simulink library "Actuator_AC_Lib"  (R2014a)
settings: Solver=ode45  StartTime=0.0  StopTime=10.0  RelTol=1e-3
undefined symbols (not defined in the file): APN_Param, DiscIntNeverNeededParam, driveGuiManager, gcbh
libraries: powerlib x14, Actuator_AC_Lib x3, AC6DriveInternalModels x3, simulink x3, DriveInternalModels x1, Lamp_Lib x1
Description:
  | Copyright 2014 The MathWorks, Inc.
settings Model: Creator=smiller  LastModifiedBy=psanghvi

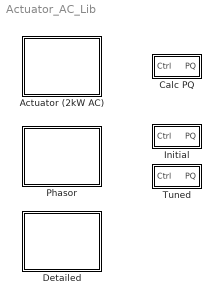
== system Actuator_AC_Lib ==
  Actuator (2kW AC) : Subsystem  BlockChoice=Detailed
      settings: TemplateBlock=self  MemberBlocks=Detailed,Phasor
  Calc PQ : Subsystem  BlockChoice=Initial
      settings: TemplateBlock=self  MemberBlocks=Initial,Tuned
  Detailed : Subsystem
      mask Display: image(imread('ActuatorAC_Detailed_IMAGE.jpg'));
  Initial : Subsystem
  Phasor : Subsystem
      mask Display: image(imread('ActuatorAC_Phasor_IMAGE.jpg'));
  Tuned : Subsystem

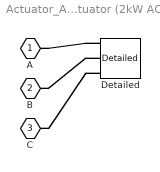
== system Actuator_AC_Lib/Actuator (2kW AC) ==
  Detailed : Actuator_AC_Lib/Detailed  SystemSampleTime=-1
  A : PMIOPort  Port=1  Side=Left
  B : PMIOPort  Port=2  Side=Left
  C : PMIOPort  Port=3  Side=Left
  connections:
  Detailed/LConn1 -- A/RConn1
  Detailed/LConn2 -- B/RConn1
  Detailed/LConn3 -- C/RConn1

== system Actuator_AC_Lib/Calc PQ ==
  Ctrl : Inport
  Initial : Actuator_AC_Lib/Initial
  PQ : Outport
  wires:
  Ctrl/1 -> Initial/1
  Initial/1 -> PQ/1

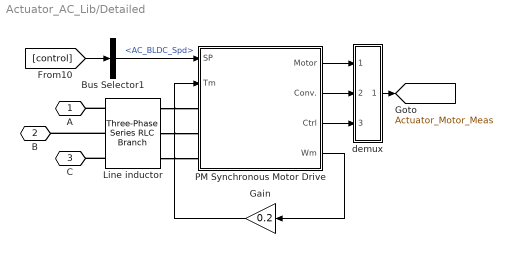
== system Actuator_AC_Lib/Detailed ==
  Bus Selector1 : BusSelector  OutputSignals=AC_BLDC_Spd
  Gain : Gain  Gain=0.2
  Line inductor : powerlib/Elements/Three-Phase Series RLC Branch  LConnTagsString=A|B|C  RConnTagsString=A|B|C  BranchType=L  Resistance=[]  Inductance=1e-3  Capacitance=[]  Measurements=None
  PM Synchronous Motor Drive : Subsystem  LoadFcn=driveGuiManager('Load',get_param(gcb,'driveType'), gcbh);  mask(PM Synchronous Motor Drive){AverageValue=on, MechanicalLoad=Torque Tm, driveType=AC6}
      mask prompts: AverageValue "Average value model"; MechanicalLoad "Mechanical input:"; driveType "Drive type:"
      mask init:
      | block = gcbh;
      | [X1,X1m,X2,X2m,X3,X4,Y1,Y1m,Y2,Y2m,Y3,Y4,color1,color2]=spsdrivelogo;
      | Ts = drivelibInitSampleTime(block);    
      | driveGuiManager('Siminit',driveType,block);
      | SetInternalDriveModel(driveType,AverageValue,block);
      | setInternalDriveMechInput(driveType,getfullname(block));
      | power_initmask();
      settings: DeleteFcn="driveGuiManager('Delete',get_param(gcb,'driveType')  ,gcbh)"  CloseFcn="driveGuiManager('Delete',get_param(gcb,'driveType')  ,gcbh)"  ParentCloseFcn="driveGuiManager('Hide',get_param(gcb,'driveType')  ,gcbh)"
      settings: OpenFcn=|
      | if (power_openblockproxy ('secondary'))
      | driveGuiManager('Create',get_param(gcb,'driveType')  ,gcbh)
      | end;
      mask Help: web(psbhelp)
      mask TypeOptions MechanicalLoad: Torque Tm | Speed w
      mask TypeOptions driveType: AC6
      mask Display:
      | patch([X1 X1m],[Y1 Y1m],color1);
      | patch(X3,Y3,color2);
      | plot([X1 X1m X2 X2m X3 X4],[Y1 Y1m Y2 Y2m Y3 Y4]);
      | text(0.5,0.3,'AC6','HorizontalAlignment','center')
  demux : Subsystem
  A : PMIOPort  Port=1  Side=Left
  B : PMIOPort  Port=2  Side=Left
  C : PMIOPort  Port=3  Side=Left
  tag scope: Actuator_Motor_Meas=global
  wires:
  PM Synchronous Motor Drive/3(Ctrl) -> demux/3(Ctrl)
  PM Synchronous Motor Drive/2(Conv.) -> demux/2(Conv.)
  PM Synchronous Motor Drive/1(Motor) -> demux/1(motor)
  PM Synchronous Motor Drive/4(Wm) -> Gain/1
  Gain/1 -> PM Synchronous Motor Drive/2(Tm)
  Bus Selector1/1 -> PM Synchronous Motor Drive/1(SP)  "<AC_BLDC_Spd>"
  demux/1(S) -> [Actuator_Motor_Meas]
  [control] -> Bus Selector1/1
  connections:
  Line inductor/LConn1 -- A/RConn1
  Line inductor/LConn2 -- B/RConn1
  Line inductor/LConn3 -- C/RConn1
  Line inductor/RConn1 -- PM Synchronous Motor Drive/LConn1
  Line inductor/RConn2 -- PM Synchronous Motor Drive/LConn2
  Line inductor/RConn3 -- PM Synchronous Motor Drive/LConn3

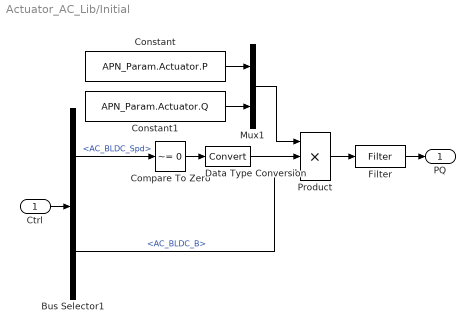
== system Actuator_AC_Lib/Initial ==
  Ctrl : Inport
  Bus Selector1 : BusSelector  OutputSignals=AC_BLDC_Spd,AC_BLDC_B
  Compare To Zero : simulink/Logic and Bit Operations/Compare To Zero  relop=~=  OutDataTypeStr=boolean
  Constant : Constant  Value=APN_Param.Actuator.P
  Constant1 : Constant  Value=APN_Param.Actuator.Q
  Data Type Conversion : DataTypeConversion
  Filter : Lamp_Lib/Initial/Filter  b=1e-2  x_initial=[APN_Param.Actuator.P APN_Param.Actuator.Q]*0
  Mux1 : Mux  Inputs=2
  Product : Product  Inputs=3
  PQ : Outport
  wires:
  Filter/1 -> PQ/1
  Bus Selector1/2 -> Product/3  "<AC_BLDC_B>"
  Bus Selector1/1 -> Compare To Zero/1  "<AC_BLDC_Spd>"
  Ctrl/1 -> Bus Selector1/1
  Compare To Zero/1 -> Data Type Conversion/1
  Data Type Conversion/1 -> Product/2
  Mux1/1 -> Product/1
  Constant/1 -> Mux1/1
  Constant1/1 -> Mux1/2
  Product/1 -> Filter/1

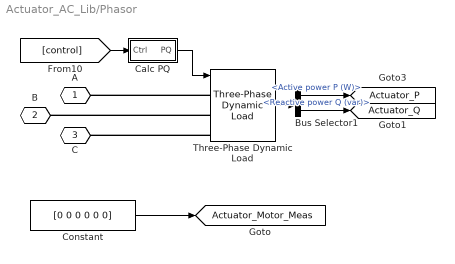
== system Actuator_AC_Lib/Phasor ==
  Bus Selector1 : BusSelector  OutputSignals=Active power P (W),Reactive power Q (var)
  Calc PQ : Subsystem  BlockChoice=Initial
      settings: AttributesFormatString=%<BlockChoice>  TemplateBlock=Actuator_AC_Lib/Calc PQ  MemberBlocks=Initial,Tuned
  Constant : Constant  Value=[0 0 0 0 0 0]
  Three-Phase Dynamic Load : powerlib/Elements/Three-Phase Dynamic Load  NominalVoltage=[ 500e3 400 ]  ActiveReactivePowers=[APN_Param.Actuator.P APN_Param.Actuator.Q]  PositiveSequence=[0.0004 0]  ExternalControl=on  NpNq=[1.3 2]  TimeConstants="[0  0  0  0]"  MinimumVoltage=0.7  LoadFlowParameters=[4,0,0,0,0]
  A : PMIOPort  Port=1  Side=Right
  B : PMIOPort  Port=2  Side=Right
  C : PMIOPort  Port=3  Side=Right
  tag scope: Actuator_Motor_Meas=global, Actuator_P=global, Actuator_Q=global
  wires:
  Bus Selector1/1 -> [Actuator_P]  "<Active power P (W)>"
  Three-Phase Dynamic Load/1 -> Bus Selector1/1
  Calc PQ/1(PQ) -> Three-Phase Dynamic Load/1
  Constant/1 -> [Actuator_Motor_Meas]
  Bus Selector1/2 -> [Actuator_Q]  "<Reactive power Q (var)>"
  [control] -> Calc PQ/1(Ctrl)
  connections:
  Three-Phase Dynamic Load/LConn3 -- C/RConn1
  Three-Phase Dynamic Load/LConn1 -- A/RConn1
  Three-Phase Dynamic Load/LConn2 -- B/RConn1

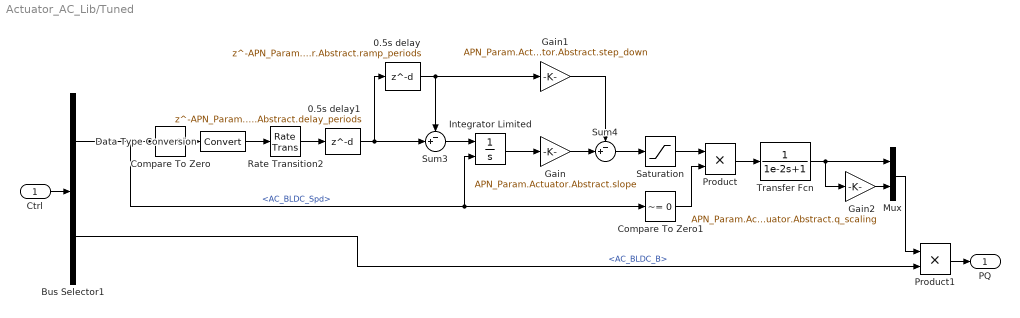
== system Actuator_AC_Lib/Tuned ==
  Ctrl : Inport
  0.5s delay : Delay  DelayLength=APN_Param.Actuator.Abstract.ramp_periods  SampleTime=0.01
  0.5s delay1 : Delay  DelayLength=APN_Param.Actuator.Abstract.delay_periods  SampleTime=0.01
  Bus Selector1 : BusSelector  OutputSignals=AC_BLDC_Spd,AC_BLDC_B
  Compare To Zero : simulink/Logic and Bit Operations/Compare To Zero  relop=~=  OutDataTypeStr=boolean
  Compare To Zero1 : simulink/Logic and Bit Operations/Compare To Zero  relop=~=  OutDataTypeStr=boolean
  Data Type Conversion : DataTypeConversion
  Gain : Gain  Gain=APN_Param.Actuator.Abstract.slope
  Gain1 : Gain  Gain=APN_Param.Actuator.Abstract.step_down
  Gain2 : Gain  Gain=APN_Param.Actuator.Abstract.q_scaling
  Integrator Limited : Integrator  ExternalReset=falling  LimitOutput=on  UpperSaturationLimit=1  LowerSaturationLimit=0
  Mux : Mux  Inputs=2
  Product : Product
  Product1 : Product
  Rate Transition2 : RateTransition  OutPortSampleTime=0.01
  Saturation : Saturate  UpperLimit=1160  LowerLimit=0
  Sum3 : Sum  Inputs=-+|  SaturateOnIntegerOverflow=on  InputSameDT=on  OutDataTypeStr=Inherit: Same as first input
  Sum4 : Sum  Inputs=-+|  SaturateOnIntegerOverflow=on  InputSameDT=on  OutDataTypeStr=Inherit: Same as first input
  Transfer Fcn : TransferFcn  Denominator=[1e-2 1]
  PQ : Outport
  wires:
  Compare To Zero1/1 -> Product/2
  Saturation/1 -> Product/1
  Sum4/1 -> Saturation/1
  0.5s delay/1 -> Gain1/1, Sum3/1
  Gain1/1 -> Sum4/1
  Product/1 -> Transfer Fcn/1
  Sum3/1 -> Integrator Limited/1
  Rate Transition2/1 -> 0.5s delay1/1
  Gain/1 -> Sum4/2
  Data Type Conversion/1 -> Rate Transition2/1
  Integrator Limited/1 -> Gain/1
  Compare To Zero/1 -> Data Type Conversion/1
  Transfer Fcn/1 -> Gain2/1, Mux/1
  Ctrl/1 -> Bus Selector1/1
  Gain2/1 -> Mux/2
  Mux/1 -> Product1/1
  Bus Selector1/1 -> Integrator Limited/2, Compare To Zero1/1, Compare To Zero/1  "<AC_BLDC_Spd>"
  0.5s delay1/1 -> Sum3/2, 0.5s delay/1
  Bus Selector1/2 -> Product1/2  "<AC_BLDC_B>"
  Product1/1 -> PQ/1

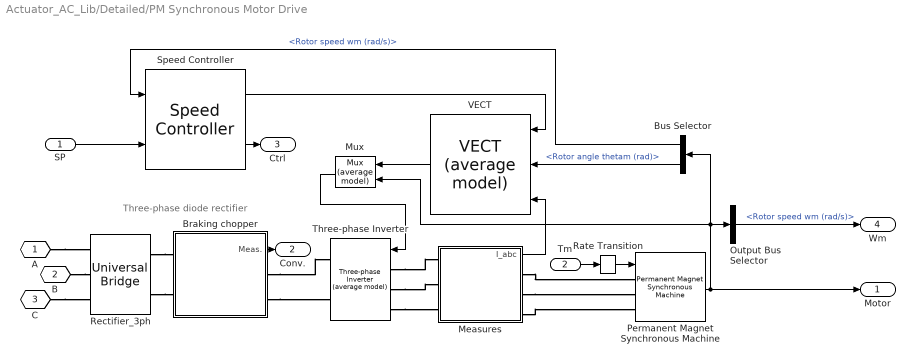
== system Actuator_AC_Lib/Detailed/PM Synchronous Motor Drive ==
  note: Three-phase
      | diode rectifier
  SP : Inport
  Tm : Inport  Port=2
  Braking chopper : Subsystem  StartFcn=|  mask(Braking chopper){chopa=290, chopd=280, freq_chop=4000, cap_bus=2000e-6, br=8}
      | chopa=str2num(get_param(gcb,'chopa'));                                                               
      | chopd=str2num(get_param(gcb,'chopd'));                                                               
      | if (chopa < chopd)                                                                                   
      |     error('Activation voltage must be greater than or equal to shutdown voltage in Braking chopper');
      | end
      mask prompts: chopa "Chopper activation voltage (V)"; chopd "Chopper shutdown voltage (V)"; freq_chop "Braking chopper frequency (Hz)"; cap_bus "DC bus capacitance (F)"; br "Braking resistance (ohms)"
      mask help: This block implement a DC link between the rectifier and the inverter. It also contains a DC bus integrated braking chopper. The braking resistor must be set properly to avoid oscillation.
      mask init:
      | if chopa < chopd;
      |     chopa = chopd;
      | end
      | [X1,X1m,X2,X2m,X3,X4,Y1,Y1m,Y2,Y2m,Y3,Y4,color1,color2]=spsdrivelogo;
      mask Display:
      | patch([X1 X1m],[Y1 Y1m],color1);
      | patch(X3,Y3,color2);
      | plot([X1 X1m X2 X2m X3 X4],[Y1 Y1m Y2 Y2m Y3 Y4]);
  Bus Selector : BusSelector  OutputSignals=Rotor speed wm (rad/s),Rotor angle thetam (rad)
  Measures : Subsystem
  Mux : AC6DriveInternalModels/Mux (average model)
  Output Bus Selector : BusSelector  OutputSignals=Rotor speed wm (rad/s)
  Permanent Magnet Synchronous Machine : powerlib/Machines/Permanent Magnet Synchronous Machine  NbPhases=3  FluxDistribution=Sinusoidal  RotorType=Round  MechanicalLoad=Torque Tm  PresetModel=No  ShowDetailedParameters=on  MeasurementBus=off  Resistance=0.2  Inductance=0  dqInductances=[8.5e-3,8.5e-3]  La=0.000835  MachineConstant=Flux linkage established by magnets (V.s)  Flux=0.175  VoltageCst=126.966  TorqueCst=1.05  Flat=0  Mechanical=[0.089,0.005,4]  PolePairs=4  InitialConditions=[0,0,0,0]  InitialConditions5ph=[0 0 0 0 0 0]  TsPowergui=0  TsBlock=-1  RefAngle=90 degrees behind phase A axis (modified Park)
      settings: AttributesFormatString=\n
  Rate Transition : RateTransition  OutPortSampleTime=Ts
  Rectifier_3ph : powerlib/Power Electronics/Universal Bridge  Arms=3  SnubberResistance=10e3  SnubberCapacitance=20e-9  Device=Diodes  Ron=1e-3  Lon=0  ForwardVoltages="[  0,  0  ]"  ForwardVoltage=1.3  GTOparameters=[ 10e-6, 20e-6 ]  IGBTparameters=[ 1e-6 , 2e-6 ]  Measurements=All voltages and currents  Measurements_2=None  converterType=Rectifier
  Speed Controller : DriveInternalModels/AC drives/Speed Controller AC67/Speed Controller  SwK=Speed regulation  ramp=[-1000,1000]  kp=5  ki=100  fc=100  ctrl_sat=[-50,50]  Tsc=150e-6
  Three-phase Inverter : AC6DriveInternalModels/Three-phase Inverter (average model)  Arms=3  SnubberResistance=5000  SnubberCapacitance=inf  Device=IGBT / Diodes  Ron=1e-3  Lon=0  ForwardVoltages=[0.8,0.8]  ForwardVoltage=0  GTOparameters=[0,0]  IGBTparameters=[1e-6,2e-6]  Measurements=All voltages and currents  converterType=Inverter  SourceFrequency=60  dqInductances=[8.5e-3,8.5e-3]  Flux=0.175  Resistance=0.2  p=4
  VECT : AC6DriveInternalModels/VECT (average model)  nb_p=4  lambda=0.175  freq_max=20e3  Ts_vect=50e-6  h=0.1
  A : PMIOPort  Port=1  Side=Left
  B : PMIOPort  Port=2  Side=Left
  C : PMIOPort  Tag=PMCPort  Port=3  Side=Left
  Motor : Outport
  Conv. : Outport  Port=2
  Ctrl : Outport  Port=3
  Wm : Outport  Port=4
  wires:
  Rate Transition/1 -> Permanent Magnet Synchronous Machine/1
  Output Bus Selector/1 -> Wm/1  "<Rotor speed wm (rad/s)>"
  Braking chopper/1(Meas.) -> Conv./1
  SP/1 -> Speed Controller/2
  Permanent Magnet Synchronous Machine/1 -> Motor/1, Mux/2, Bus Selector/1, Output Bus Selector/1
  Measures/1(I_abc) -> VECT/3
  Speed Controller/1 -> VECT/1
  Tm/1 -> Rate Transition/1
  Speed Controller/2 -> Ctrl/1
  VECT/1 -> Mux/1
  Mux/1 -> Three-phase Inverter/1
  Bus Selector/1 -> Speed Controller/1  "<Rotor speed wm (rad/s)>"
  Bus Selector/2 -> VECT/2  "<Rotor angle thetam (rad)>"
  connections:
  Braking chopper/RConn1 -- Three-phase Inverter/RConn1
  Rectifier_3ph/RConn2 -- Braking chopper/LConn2
  Rectifier_3ph/RConn1 -- Braking chopper/LConn1
  A/RConn1 -- Rectifier_3ph/LConn1
  Braking chopper/RConn2 -- Three-phase Inverter/RConn2
  Measures/RConn1 -- Permanent Magnet Synchronous Machine/LConn1
  Measures/RConn2 -- Permanent Magnet Synchronous Machine/LConn2
  Measures/RConn3 -- Permanent Magnet Synchronous Machine/LConn3
  B/RConn1 -- Rectifier_3ph/LConn2
  C/RConn1 -- Rectifier_3ph/LConn3
  Three-phase Inverter/LConn1 -- Measures/LConn1
  Three-phase Inverter/LConn2 -- Measures/LConn2
  Three-phase Inverter/LConn3 -- Measures/LConn3

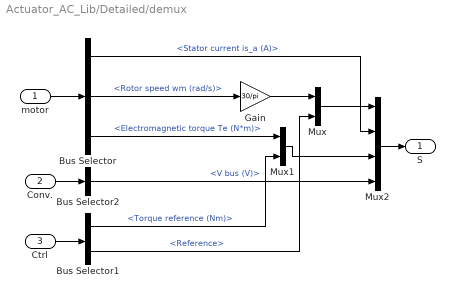
== system Actuator_AC_Lib/Detailed/demux ==
  motor : Inport
  Conv. : Inport  Port=2
  Ctrl : Inport  Port=3
  Bus Selector : BusSelector  OutputSignals=Stator current is_a (A),Rotor speed wm (rad/s),Electromagnetic torque Te (N*m)
  Bus Selector1 : BusSelector  OutputSignals=Torque reference (Nm),Reference
  Bus Selector2 : BusSelector  OutputSignals=V bus (V)
  Gain : Gain  Gain=30/pi  SaturateOnIntegerOverflow=on  OutDataTypeStr=Inherit: Same as input  ParamDataTypeStr=Inherit: Same as input
  Mux : Mux  Inputs=2
  Mux1 : Mux  Inputs=2
  Mux2 : Mux
  S : Outport
  wires:
  motor/1 -> Bus Selector/1
  Mux/1 -> Mux2/2
  Mux1/1 -> Mux2/3
  Bus Selector/3 -> Mux1/1  "<Electromagnetic torque Te (N*m)>"
  Bus Selector/1 -> Mux2/1  "<Stator current is_a (A)>"
  Gain/1 -> Mux/1
  Bus Selector1/2 -> Mux/2  "<Reference>"
  Bus Selector1/1 -> Mux1/2  "<Torque reference (Nm)>"
  Ctrl/1 -> Bus Selector1/1
  Conv./1 -> Bus Selector2/1
  Bus Selector2/1 -> Mux2/4  "<V bus (V)>"
  Bus Selector/2 -> Gain/1  "<Rotor speed wm (rad/s)>"
  Mux2/1 -> S/1

== system Actuator_AC_Lib/Phasor/Calc PQ ==
  Ctrl : Inport
  Initial : Actuator_AC_Lib/Initial
  PQ : Outport
  wires:
  Ctrl/1 -> Initial/1
  Initial/1 -> PQ/1

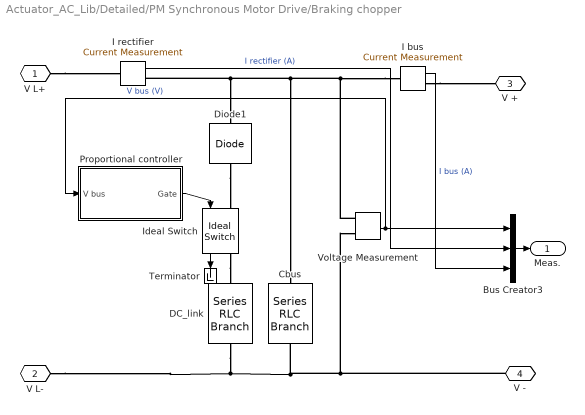
== system Actuator_AC_Lib/Detailed/PM Synchronous Motor Drive/Braking chopper ==
  Bus Creator3 : BusCreator  Inputs=3
  Cbus : powerlib/Elements/Series RLC Branch  LConnTagsString=__new0  RConnTagsString=__new0  BranchType=C  Resistance=[]  Inductance=[]  SetiL0=off  InitialCurrent=0  Capacitance=cap_bus  Setx0=on  InitialVoltage=300  Measurements=None
  DC_link : powerlib/Elements/Series RLC Branch  LConnTagsString=__new0  RConnTagsString=__new0  BranchType=R  Resistance=br  Inductance=[]  SetiL0=off  InitialCurrent=0  Capacitance=[]  Setx0=off  InitialVoltage=0  Measurements=None
  Diode1 : powerlib/Power Electronics/Diode  Ron=1e-3  Lon=0  Vf=0.8  IC=0  UseSnubber=off  Rs=10e3  Cs=inf  Measurements=off
  I bus : powerlib/Measurements/Current Measurement  PhasorSimulation=off  OutputType=Complex  PSBequivalent=0
  I rectifier : powerlib/Measurements/Current Measurement  PhasorSimulation=off  OutputType=Complex  PSBequivalent=0
  Ideal Switch : powerlib/Power Electronics/Ideal Switch  Ron=1e-3  Lon=0  IC=0  Rs=10e3  Cs=inf  Measurements=on
      settings: AttributesFormatString=\n
  Proportional controller : Subsystem
  Terminator : Terminator
  Voltage Measurement : powerlib/Measurements/Voltage Measurement  Tag=PoWeRsYsTeMmEaSuReMeNt  PhasorSimulation=off  OutputType=Complex  PSBequivalent=0
  V L+ : PMIOPort  Port=1  Side=Left
  V L- : PMIOPort  Port=2  Side=Left
  V + : PMIOPort  Port=3  Side=Right
  V - : PMIOPort  Port=4  Side=Right
  Meas. : Outport
  wires:
  I bus/1 -> Bus Creator3/3  "I bus (A)"
  I rectifier/1 -> Bus Creator3/2  "I rectifier (A)"
  Bus Creator3/1 -> Meas./1
  Proportional controller/1(Gate) -> Ideal Switch/1
  Voltage Measurement/1 -> Bus Creator3/1, Proportional controller/1(V bus)  "V bus (V)"
  Ideal Switch/1 -> Terminator/1
  connections:
  V L+/RConn1 -- I rectifier/LConn1
  I bus/RConn1 -- V +/RConn1
  Diode1/RConn1 -- Ideal Switch/LConn1
  I bus/LConn1 -- Voltage Measurement/LConn1 -- Cbus/LConn1 -- I rectifier/RConn1 -- Diode1/LConn1
  Cbus/RConn1 -- DC_link/RConn1 -- V L-/RConn1 -- Voltage Measurement/LConn2 -- V -/RConn1
  Ideal Switch/RConn1 -- DC_link/LConn1

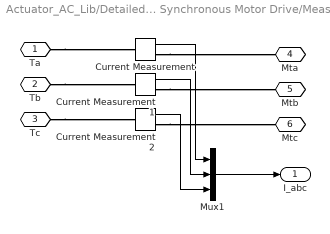
== system Actuator_AC_Lib/Detailed/PM Synchronous Motor Drive/Measures ==
  Current Measurement : powerlib/Measurements/Current Measurement  Tag=PoWeRsYsTeMmEaSuReMeNt  PhasorSimulation=off  OutputType=Magnitude  PSBequivalent=0
  Current Measurement1 : powerlib/Measurements/Current Measurement  Tag=PoWeRsYsTeMmEaSuReMeNt  PhasorSimulation=off  OutputType=Magnitude  PSBequivalent=0
  Current Measurement2 : powerlib/Measurements/Current Measurement  Tag=PoWeRsYsTeMmEaSuReMeNt  PhasorSimulation=off  OutputType=Magnitude  PSBequivalent=0
  Mux1 : Mux  Inputs=3
  Ta : PMIOPort  Port=1  Side=Left
  Tb : PMIOPort  Port=2  Side=Left
  Tc : PMIOPort  Port=3  Side=Left
  Mta : PMIOPort  Port=4  Side=Right
  Mtb : PMIOPort  Port=5  Side=Right
  Mtc : PMIOPort  Port=6  Side=Right
  I_abc : Outport
  wires:
  Mux1/1 -> I_abc/1
  Current Measurement2/1 -> Mux1/3
  Current Measurement/1 -> Mux1/1
  Current Measurement1/1 -> Mux1/2
  connections:
  Current Measurement2/RConn1 -- Mtc/RConn1
  Tc/RConn1 -- Current Measurement2/LConn1
  Ta/RConn1 -- Current Measurement/LConn1
  Current Measurement/RConn1 -- Mta/RConn1
  Tb/RConn1 -- Current Measurement1/LConn1
  Current Measurement1/RConn1 -- Mtb/RConn1

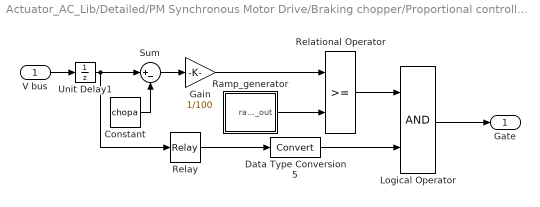
== system Actuator_AC_Lib/Detailed/PM Synchronous Motor Drive/Braking chopper/Proportional controller ==
  V bus : Inport
  Constant : Constant  Value=chopa
  Data Type Conversion5 : DataTypeConversion  SaturateOnIntegerOverflow=on  RndMeth=Zero
  Gain : Gain  Gain=1/100  SaturateOnIntegerOverflow=on  OutDataTypeStr=Inherit: Same as input  ParamDataTypeStr=Inherit: Same as input
  Logical Operator : Logic
  Ramp_generator : Subsystem
  Relational Operator : RelationalOperator  InputSameDT=on
  Relay : Relay  OnSwitchValue=chopa  OffSwitchValue=chopd
  Sum : Sum  Inputs=|+-  SaturateOnIntegerOverflow=on  InputSameDT=on  OutDataTypeStr=Inherit: Same as first input
  Unit Delay1 : UnitDelay  SampleTime=Ts
  Gate : Outport
  wires:
  Ramp_generator/1(ramp_out) -> Relational Operator/2
  Unit Delay1/1 -> Sum/1, Relay/1
  Sum/1 -> Gain/1
  Gain/1 -> Relational Operator/1
  Constant/1 -> Sum/2
  V bus/1 -> Unit Delay1/1
  Relational Operator/1 -> Logical Operator/1
  Logical Operator/1 -> Gate/1
  Relay/1 -> Data Type Conversion5/1
  Data Type Conversion5/1 -> Logical Operator/2

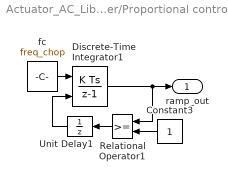
== system Actuator_AC_Lib/Detailed/PM Synchronous Motor Drive/Braking chopper/Proportional controller/Ramp_generator ==
  Constant3 : Constant
  Discrete-Time Integrator1 : DiscreteIntegrator  ExternalReset=rising  SampleTime=Ts  ICPrevOutput=DiscIntNeverNeededParam  ICPrevScaledInput=DiscIntNeverNeededParam
  Relational Operator1 : RelationalOperator  InputSameDT=on
  Unit Delay1 : UnitDelay  SampleTime=Ts
  fc : Constant  Value=freq_chop
  ramp_out : Outport
  wires:
  fc/1 -> Discrete-Time Integrator1/1
  Discrete-Time Integrator1/1 -> Relational Operator1/1, ramp_out/1
  Constant3/1 -> Relational Operator1/2
  Relational Operator1/1 -> Unit Delay1/1
  Unit Delay1/1 -> Discrete-Time Integrator1/2
